simulink model "Final_Model_Project1"  (R2023b)
settings: Solver=ode4  StartTime=0.0  StopTime=2  FixedStep=2e-6  RelTol=1e-3
values from neighbouring files (symbols this model uses):
  C1 = 0.7029    [Fixed_Speed_Wind_Turbine.m]
  C2 = 116.055    [Fixed_Speed_Wind_Turbine.m]
  C3 = 0.4    [Fixed_Speed_Wind_Turbine.m]
  C4 = 0    [Fixed_Speed_Wind_Turbine.m]
  C5 = 8.6614    [Fixed_Speed_Wind_Turbine.m]
  C6 = 21.5    [Fixed_Speed_Wind_Turbine.m]
  C7 = 0.00684    [Fixed_Speed_Wind_Turbine.m]
  Fg = 50    [Fixed_Speed_Wind_Turbine.m]
  Fs = 50    [Fixed_Speed_Wind_Turbine.m]
  J = 1200    [Fixed_Speed_Wind_Turbine.m]
  Llr = 0.06492e-3    (= 6.492e-05)    [Fixed_Speed_Wind_Turbine.m]
  Lls = 0.06492e-3    (= 6.492e-05)    [Fixed_Speed_Wind_Turbine.m]
  optical_tsr_value = (n_mr*(2*pi/60)*r_t)/v_wr    (= 6.49262481742)    [Fixed_Speed_Wind_Turbine.m]
  P = 2    [Fixed_Speed_Wind_Turbine.m]
  p_row = 1.225    [Fixed_Speed_Wind_Turbine.m]
  Ps = (2.3e6)    (= 2300000)    [Fixed_Speed_Wind_Turbine.m]
  r_t = 46.5    [Fixed_Speed_Wind_Turbine.m]
  rgb = 94.5    [Fixed_Speed_Wind_Turbine.m]
  Rr = 1.497e-3    (= 0.001497)    [Fixed_Speed_Wind_Turbine.m]
  Rs = 1.102e-3    (= 0.001102)    [Fixed_Speed_Wind_Turbine.m]
  slip = (nsyn-nmInit)/nsyn    (= 0.0333333333333)    [Fixed_Speed_Wind_Turbine.m]
  SR = 2.59e6    (= 2590000)    [Fixed_Speed_Wind_Turbine.m]
  VgLL = 690    [Fixed_Speed_Wind_Turbine.m]
  VsLL = 690    [Fixed_Speed_Wind_Turbine.m]
libraries: spsAsynchronousMachineSIUnitsLib x1, spsThreePhaseVIMeasurementLib x1, slpidlib x1, spsPower3phInstantaneousLib x1, spsGroundLib x1, spsThreePhaseProgrammableVoltageSourceLib x1, simulink x1, sps_lib x1
settings Model: Creator=priya  LastModifiedBy=priya
settings SolverCC: AutoInsertRateTranBlk=on

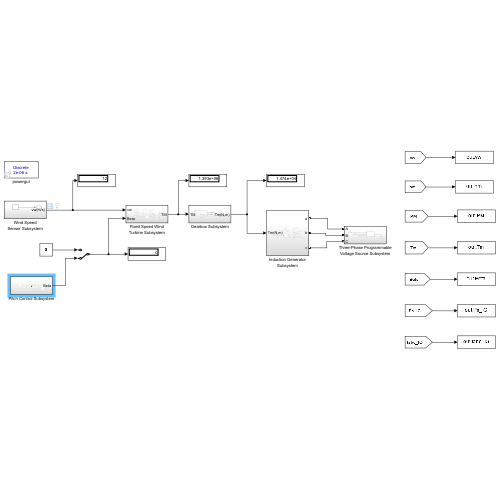
[thumbnail: Simulink's stored preview of the top-level diagram]
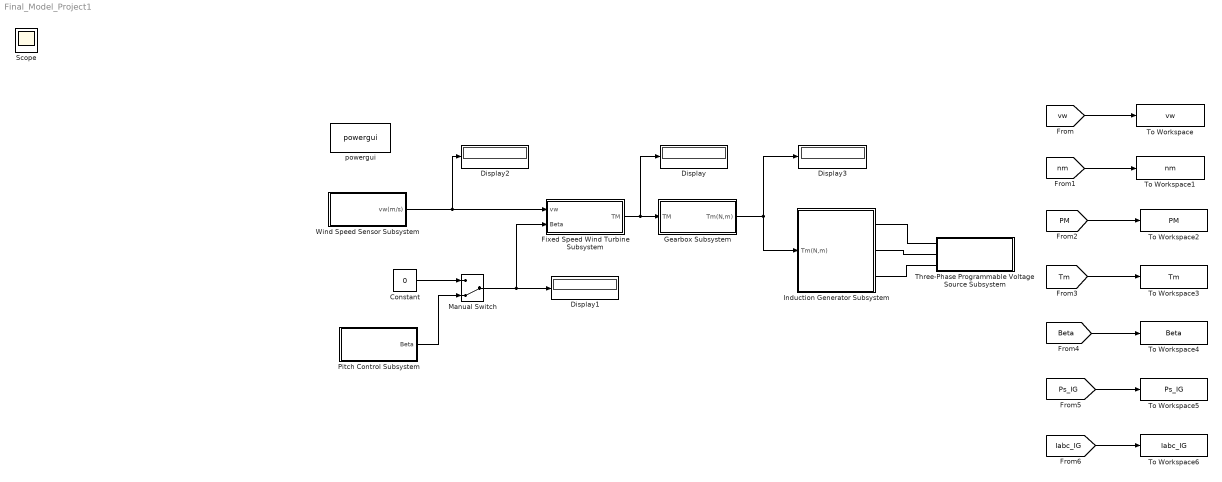
== system Final_Model_Project1 ==
  Constant : Constant  Value=0
  Display{,1..3} (4 alike) : Display
  Fixed Speed Wind Turbine Subsystem : Subsystem
  Gearbox Subsystem : Subsystem
  Induction Generator Subsystem : Subsystem
  Manual Switch : ManualSwitch  CurrentSetting=0
  Pitch Control Subsystem : Subsystem
  Three-Phase Programmable Voltage Source Subsystem : Subsystem
  To Workspace : ToWorkspace  VariableName=vw  SampleTime=-1
  To Workspace1 : ToWorkspace  VariableName=nm  SampleTime=-1
  To Workspace2 : ToWorkspace  VariableName=PM  SampleTime=-1
  To Workspace3 : ToWorkspace  VariableName=Tm  SampleTime=-1
  To Workspace4 : ToWorkspace  VariableName=Beta  SampleTime=-1
  To Workspace5 : ToWorkspace  VariableName=Ps_IG  SampleTime=-1
  To Workspace6 : ToWorkspace  VariableName=Iabc_IG  SampleTime=-1
  Wind Speed Sensor Subsystem : Subsystem
  powergui : sps_lib/powergui  Priority=1  SimulationMode=Discrete  SampleTime=2e-6  frequency=60  Iterations=50  frequencyindice=50  Pbase=100e6  ErrMax=1e-4  UnitsV=kV  UnitsW=MW  buscounter=0  FunctionMessages=off  echomessages=off  EnableUseOfTLC=off  CurrentSourceSwitches=off  DisableSnubberDevices=off  DisableRonSwitches=off  DisableVfSwitches=off  DisplayEquations=off  AutomaticDiscreteSolvers=off  SolverType=Tustin/Backward Euler (TBE)  Interpol=off  ExternalGateDelay=off  methode=off  Ts=100  x0status=blocks  SPID=on  SwTol=0  HookPort=off  NonlinearTolerance=1e-4  nMaxIteration=100  ContinueOnMaxIteration=off  RestoreLinks=warning  ResistiveCurrentMeasurement=off  Frange=[0:2:500]  Ylog=off  Xlog=on  ShowGrid=off  save=off  variable=ZData  structure=0  ZoomFFT=off  StartTime=0.0  cycles=1  DisplayStyle=1  fundamental=60  FreqAxis=off  MaxFrequency=1000  frequencyindicesteady=1  RmsSteady=1  display=off
  Scope : Scope
  wires:
  Gearbox Subsystem/1(Tm(N,m)) -> Display3/1, Induction Generator Subsystem/1(Tm(N,m))
  Pitch Control Subsystem/1(Beta) -> Manual Switch/2
  Fixed Speed Wind Turbine Subsystem/1(TM) -> Display/1, Gearbox Subsystem/1(TM)
  Manual Switch/1 -> Display1/1, Fixed Speed Wind Turbine Subsystem/2(Beta)
  Constant/1 -> Manual Switch/1
  Wind Speed Sensor Subsystem/1(vw(m/s)) -> Display2/1, Fixed Speed Wind Turbine Subsystem/1(vw)
  [vw] -> To Workspace/1
  [nm] -> To Workspace1/1
  [PM] -> To Workspace2/1
  [Tm] -> To Workspace3/1
  [Beta] -> To Workspace4/1
  [Ps_IG] -> To Workspace5/1
  [Iabc_IG] -> To Workspace6/1
  connections:
  Three-Phase Programmable Voltage Source Subsystem/LConn1 -- Induction Generator Subsystem/RConn1
  Three-Phase Programmable Voltage Source Subsystem/LConn2 -- Induction Generator Subsystem/RConn2
  Three-Phase Programmable Voltage Source Subsystem/LConn3 -- Induction Generator Subsystem/RConn3

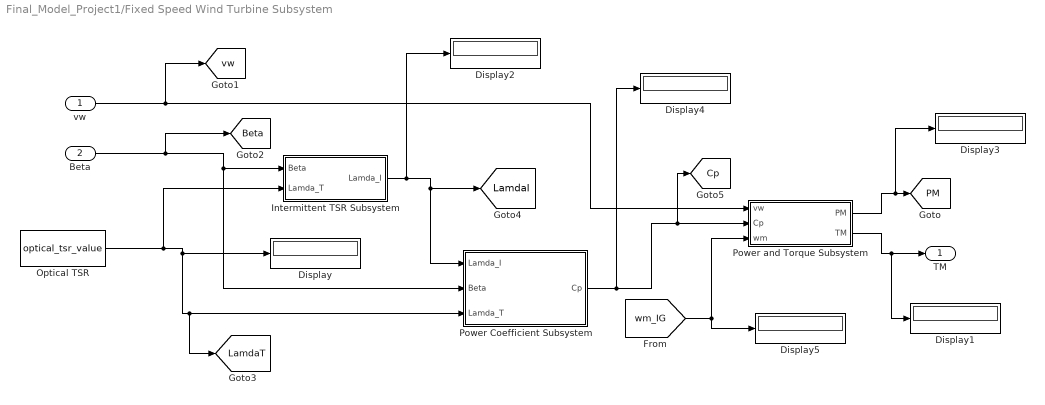
== system Final_Model_Project1/Fixed Speed Wind Turbine Subsystem ==
  vw : Inport
  Beta : Inport  Port=2
  Display{,1..5} (6 alike) : Display
  Intermittent TSR Subsystem : Subsystem
  Optical TSR : Constant  Value=optical_tsr_value
  Power Coefficient Subsystem : Subsystem
  Power and Torque Subsystem : Subsystem
  TM : Outport
  tag scope: Beta=global, Cp=global, LamdaI=global, LamdaT=global, PM=global, vw=global
  wires:
  Power and Torque Subsystem/1(PM) -> Display3/1, [PM]
  Power and Torque Subsystem/2(TM) -> Display1/1, TM/1
  Power Coefficient Subsystem/1(Cp) -> Display4/1, [Cp], Power and Torque Subsystem/2(Cp)
  Optical TSR/1 -> Intermittent TSR Subsystem/2(Lamda_T), [LamdaT], Power Coefficient Subsystem/3(Lamda_T), Display/1
  Beta/1 -> [Beta], Intermittent TSR Subsystem/1(Beta), Power Coefficient Subsystem/2(Beta)
  Intermittent TSR Subsystem/1(Lamda_I) -> Display2/1, Power Coefficient Subsystem/1(Lamda_I), [LamdaI]
  vw/1 -> [vw], Power and Torque Subsystem/1(vw)
  [wm_IG] -> Display5/1, Power and Torque Subsystem/3(wm)

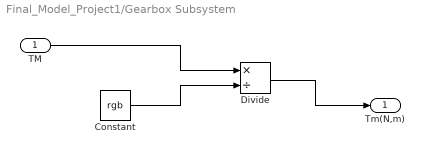
== system Final_Model_Project1/Gearbox Subsystem ==
  TM : Inport
  Constant : Constant  Value=rgb
  Divide : Product  Inputs=*/
  Tm(N,m) : Outport
  wires:
  TM/1 -> Divide/1
  Constant/1 -> Divide/2
  Divide/1 -> Tm(N,m)/1

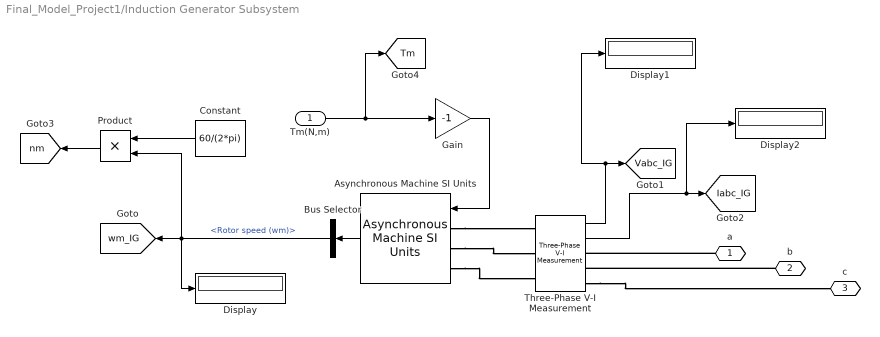
== system Final_Model_Project1/Induction Generator Subsystem ==
  Tm(N,m) : Inport
  Asynchronous Machine SI Units : spsAsynchronousMachineSIUnitsLib/Asynchronous Machine SI Units  RotorType=Squirrel-cage  PresetModel=No  MechanicalLoad=Torque Tm  ShowDetailedParameters=on  ReferenceFrame=Stationary  Units=SI  MeasurementBus=off  NominalParameters="[SR  VsLL Fs]"  VoltageRatio=1  Stator=[Rs Lls]  Rotor=[Rr Llr]  Cage1=[0.4155 0.002066]  Cage2=[0.4168 0.0003495]  Lm=Lm  Mechanical=[J 0 P]  PolePairs=2  InitialConditions=[slip 0 0 0 0 0 0 0]  SimulateSaturation=off  Saturation=[14.03593122, 27.81365428, 53.79336849, 72.68890987, 97.98006896, 148.6815601, 215.7428561, 302.9841135, 428.7778367 ; 230, 322, 414, 460, 506, 552, 598, 644, 690]  LoadFlowParameters=1492000  TsPowergui=0  TsBlock=-1  IterativeModel=Trapezoidal non iterative  IterativeDiscreteModel=Trapezoidal non iterative  Pmec=1.492e+006
  Bus Selector : BusSelector  OutputSignals=Mechanical.Rotor speed (wm)
  Constant : Constant  Value=60/(2*pi)
  Display : Display
  Display1 : Display
  Display2 : Display
  Gain : Gain  Gain=-1
  Product : Product
  Three-Phase V-I Measurement : spsThreePhaseVIMeasurementLib/Three-Phase V-I Measurement  VoltageMeasurement=phase-to-ground  SetLabelV=off  LabelV=Vabc_IG  Vpu=off  VpuLL=off  CurrentMeasurement=yes  SetLabelI=off  LabelI=Iabc_IG  Ipu=off  Pbase=100e6  Vbase=500e3  OutputType=Complex  PhasorSimulation=off  PSBequivalent=0
  a : PMIOPort  Side=Right
  b : PMIOPort  Port=2  Side=Right
  c : PMIOPort  Port=3  Side=Right
  tag scope: Iabc_IG=global, Tm=global, Vabc_IG=global, nm=global, wm_IG=global
  wires:
  Asynchronous Machine SI Units/1 -> Bus Selector/1
  Tm(N,m)/1 -> [Tm], Gain/1
  Gain/1 -> Asynchronous Machine SI Units/1
  Bus Selector/1 -> Product/2, Display/1, [wm_IG]  "<Rotor speed (wm)>"
  Three-Phase V-I Measurement/1 -> Display1/1, [Vabc_IG]
  Three-Phase V-I Measurement/2 -> Display2/1, [Iabc_IG]
  Constant/1 -> Product/1
  Product/1 -> [nm]
  connections:
  Asynchronous Machine SI Units/LConn1 -- Three-Phase V-I Measurement/LConn1
  Asynchronous Machine SI Units/LConn2 -- Three-Phase V-I Measurement/LConn2
  Asynchronous Machine SI Units/LConn3 -- Three-Phase V-I Measurement/LConn3
  Three-Phase V-I Measurement/RConn3 -- c/RConn1
  b/RConn1 -- Three-Phase V-I Measurement/RConn2
  a/RConn1 -- Three-Phase V-I Measurement/RConn1

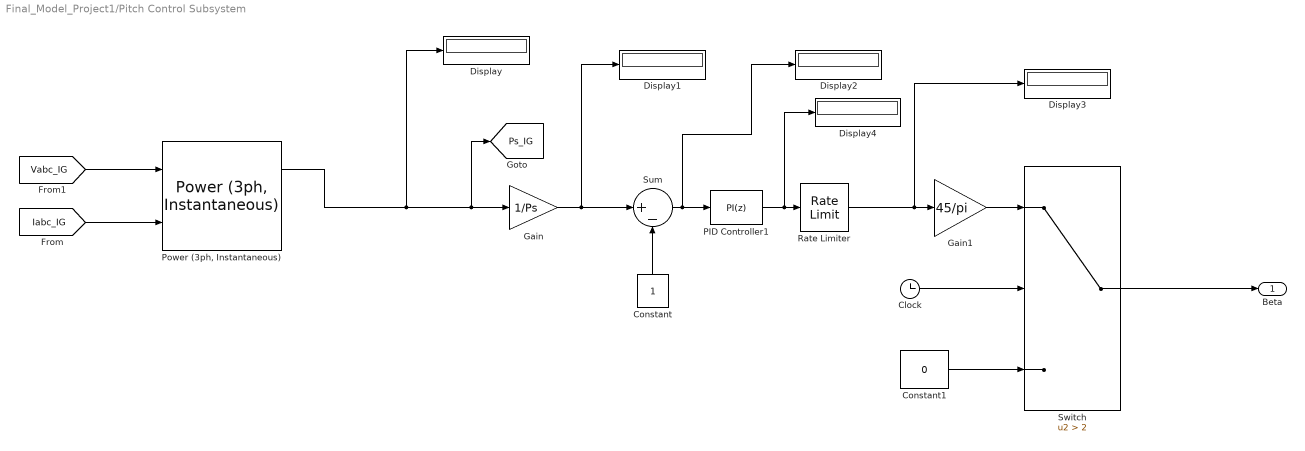
== system Final_Model_Project1/Pitch Control Subsystem ==
  Clock : Clock
  Constant : Constant
  Constant1 : Constant  Value=0
  Display{,1..4} (5 alike) : Display
  Gain : Gain  Gain=1/Ps
  Gain1 : Gain  Gain=45/pi
  PID Controller1 : slpidlib/PID Controller  Controller=PI  Form=Parallel  TimeDomain=Discrete-time  UseExternalTs=off  SampleTime=2e-6  IntegratorMethod=Forward Euler  FilterMethod=Forward Euler  ControllerParametersSource=internal  P=100  I=0.001  UseKiTs=off  D=0  N=100  UseFilter=on  TunerSelectOption=Transfer Function Based (PID Tuner App)  InitialConditionSource=internal  InitialConditionForIntegrator=0  InitialConditionForFilter=0  DifferentiatorICPrevScaledInput=0  ExternalReset=none  TrackingMode=off  Kt=1  LimitOutput=on  SatLimitsSource=internal  UpperSaturationLimit=45  LowerSaturationLimit=0  LinearizeAsGain=on  AntiWindupMode=none  Kb=1  LimitIntegrator=off  UpperIntegratorSaturationLimit=inf  LowerIntegratorSaturationLimit=-inf  POutMin=[]  POutMax=[]  IOutMin=[]  IOutMax=[]  DOutMin=[]  DOutMax=[]  NOutMin=[]  NOutMax=[]  SumOutMin=[]  SumOutMax=[]  SaturationOutMin=[]  SaturationOutMax=[]  PParamMin=[]  PParamMax=[]  IParamMin=[]  IParamMax=[]  DParamMin=[]  DParamMax=[]  NParamMin=[]  NParamMax=[]  KbParamMin=[]  KbParamMax=[]  KtParamMin=[]  KtParamMax=[]  KbOutMin=[]  KbOutMax=[]  KtOutMin=[]  KtOutMax=[]  IntegratorOutMin=[]  IntegratorOutMax=[]  FilterOutMin=[]  FilterOutMax=[]  SumI1OutMin=[]  SumI1OutMax=[]  SumI2OutMin=[]  SumI2OutMax=[]  SumI3OutMin=[]  SumI3OutMax=[]  SumI4OutMin=[]  SumI4OutMax=[]  SumDOutMin=[]  SumDOutMax=[]  DifferentiatorOutMin=[]  DifferentiatorOutMax=[]  FilterDiffOutCoefMin=[]  FilterDiffOutCoefMax=[]  ReciprocalOutMin=[]  ReciprocalOutMax=[]  SumDenOutMin=[]  SumDenOutMax=[]  SumNumOutMin=[]  SumNumOutMax=[]  DivideOutMin=[]  DivideOutMax=[]  UdiffTsProdOutMin=[]  UdiffTsProdOutMax=[]  NTsProdOutMin=[]  NTsProdOutMax=[]  UintegralTsProdOutMin=[]  UintegralTsProdOutMax=[]  UngainTsProdOutMin=[]  UngainTsProdOutMax=[]  ClampingZeroOutDataTypeStr=Inherit: Inherit via back propagation  ClampingZeroOutMin=[]  ClampingZeroOutMax=[]  FilterDenConstantOutDataTypeStr=Inherit: Inherit via back propagation  FilterDenConstantOutMin=[]  FilterDenConstantOutMax=[]  PCopyOutDataTypeStr=Inherit: Inherit via back propagation  PCopyOutMin=[]  PCopyOutMax=[]  NCopyOutDataTypeStr=Inherit: Inherit via back propagation  NCopyOutMin=[]  NCopyOutMax=[]  IntegratorContinuousStateAttributes=''  IntegratorStateMustResolveToSignalObject=off  IntegratorRTWStateStorageClass=Auto  FilterContinuousStateAttributes=''  FilterStateMustResolveToSignalObject=off  FilterRTWStateStorageClass=Auto  ParallelPVariant=InternalParameters  IdealPVariant=Disabled  IVariant=InternalParameters  DVariant=Disabled  IntegratorVariant=Discrete  SatVariant=Enabled  AWVariant=Passthrough  PCopyVariant=Disabled  TRVariant=Disabled  FdbkBlocksVariant=Forward  IdealPFdbkVariant=Disabled  SatFdbkVariant=Disabled  DerivativeFilterVariant=Disabled  NVariant=Disabled  NCopyVariant=Disabled_SignalSpec  FilterICVariant=Disabled  IntegratorICVariant=InternalICs  ExternalResetVariant=Disabled  TRSumVariant=Passthrough  SumFdbkVariant=Disabled  SumVariant=Sum_PI  TsampFilterVariant=InternalTs  TsampNgainVariant=Passthrough  TsampIntegralVariant=Disabled_SignalSpec  ExternalSaturationOutDataTypeStr=Inherit: Same as second input
  "Power (3ph, Instantaneous)" : spsPower3phInstantaneousLib/Power (3ph, Instantaneous)
  Rate Limiter : RateLimiter  RisingSlewLimit=10  FallingSlewLimit=-10  SampleTimeMode=inherited
  Sum : Sum  Inputs=|+-
  Switch : Switch  Criteria=u2 > Threshold  Threshold=2  SaturateOnIntegerOverflow=off  InputSameDT=off
  Beta : Outport
  tag scope: Ps_IG=global
  wires:
  [Vabc_IG] -> "Power (3ph, Instantaneous)"/1
  [Iabc_IG] -> "Power (3ph, Instantaneous)"/2
  "Power (3ph, Instantaneous)"/1 -> Display/1, Gain/1, [Ps_IG]
  Constant/1 -> Sum/2
  Rate Limiter/1 -> Display3/1, Gain1/1
  Gain1/1 -> Switch/1
  Clock/1 -> Switch/2
  Constant1/1 -> Switch/3
  Switch/1 -> Beta/1
  Sum/1 -> PID Controller1/1, Display2/1
  Gain/1 -> Display1/1, Sum/1
  PID Controller1/1 -> Display4/1, Rate Limiter/1

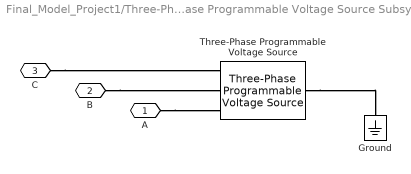
== system Final_Model_Project1/Three-Phase Programmable Voltage Source Subsystem ==
  Ground : spsGroundLib/Ground  LConnTagsString=a
  Three-Phase Programmable Voltage Source : spsThreePhaseProgrammableVoltageSourceLib/Three-Phase Programmable Voltage Source  PositiveSequence=[VgLL 0 Fg]  VariationEntity=None  VariationType=Table of time-amplitude pairs  VariationTypeAlt=Step  VariationStep=0.5  VariationRate=10  VariationMagnitude=0.3  VariationFrequency=2  VariationTiming=[1 2]  VariationPhaseA=off  Amplitudes=[1 0.8 1.2 1.0]  TimeValues=[0 0.1 0.15 0.2]  HarmonicGeneration=off  HarmonicA=[3 0.2 -25 0]  HarmonicB=[2 0.15 35 2]  Timing="[0.05  3]"  BusType=swing  Pref=0  Qref=0  Qmin=-inf  Qmax=inf
  A : PMIOPort  Side=Left
  B : PMIOPort  Port=2  Side=Left
  C : PMIOPort  Port=3  Side=Left
  connections:
  Three-Phase Programmable Voltage Source/LConn1 -- Ground/LConn1
  A/RConn1 -- Three-Phase Programmable Voltage Source/RConn1
  B/RConn1 -- Three-Phase Programmable Voltage Source/RConn2
  C/RConn1 -- Three-Phase Programmable Voltage Source/RConn3

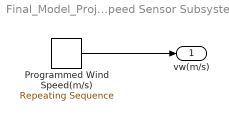
== system Final_Model_Project1/Wind Speed Sensor Subsystem ==
  Programmed Wind Speed(m/s) : simulink/Sources/Repeating Sequence  rep_seq_t=[0 1.2 2.4 2.8 3.2 3.6 5]  rep_seq_y=[0.0001 12 12 15 15 12 12]
  vw(m/s) : Outport
  wires:
  Programmed Wind Speed(m/s)/1 -> vw(m/s)/1

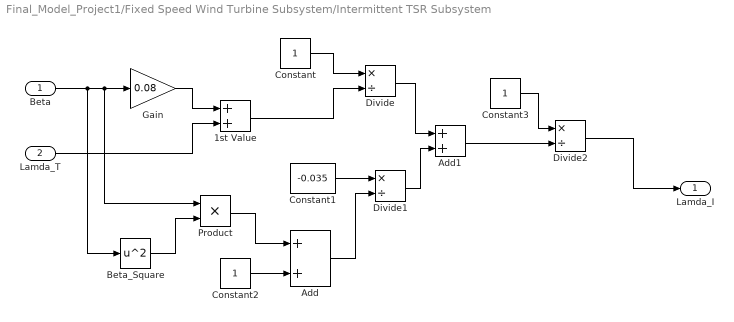
== system Final_Model_Project1/Fixed Speed Wind Turbine Subsystem/Intermittent TSR Subsystem ==
  Beta : Inport
  Lamda_T : Inport  Port=2
  1st Value : Sum
  Add : Sum
  Add1 : Sum
  Beta_Square : Math  Operator=square
  Constant : Constant
  Constant1 : Constant  Value=-0.035
  Constant2 : Constant
  Constant3 : Constant
  Divide : Product  Inputs=*/
  Divide1 : Product  Inputs=*/
  Divide2 : Product  Inputs=*/
  Gain : Gain  Gain=0.08
  Product : Product
  Lamda_I : Outport
  wires:
  Beta/1 -> Product/1, Gain/1, Beta_Square/1
  Gain/1 -> 1st Value/1
  Lamda_T/1 -> 1st Value/2
  Constant/1 -> Divide/1
  1st Value/1 -> Divide/2
  Beta_Square/1 -> Product/2
  Product/1 -> Add/1
  Constant2/1 -> Add/2
  Constant1/1 -> Divide1/1
  Add/1 -> Divide1/2
  Divide/1 -> Add1/1
  Divide1/1 -> Add1/2
  Add1/1 -> Divide2/2
  Constant3/1 -> Divide2/1
  Divide2/1 -> Lamda_I/1

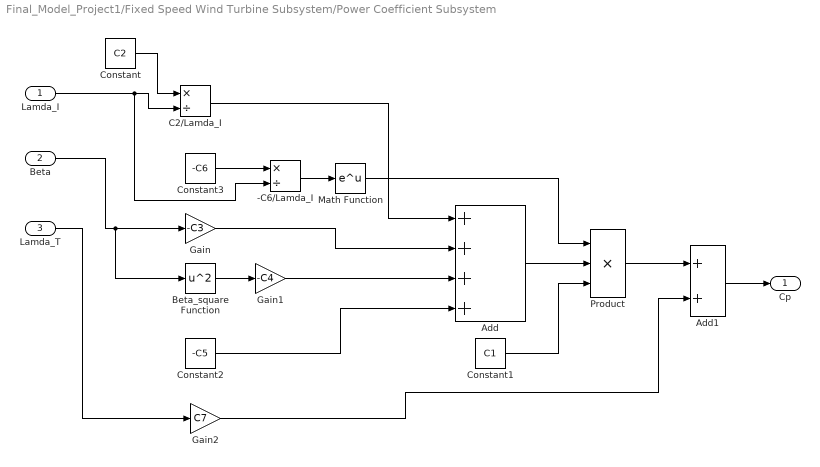
== system Final_Model_Project1/Fixed Speed Wind Turbine Subsystem/Power Coefficient Subsystem ==
  Lamda_I : Inport
  Beta : Inport  Port=2
  Lamda_T : Inport  Port=3
  -C6/Lamda_I : Product  Inputs=*/
  Add : Sum  Inputs=++++
  Add1 : Sum
  Beta_square Function : Math  Operator=square
  C2/Lamda_I : Product  Inputs=*/
  Constant : Constant  Value=C2
  Constant1 : Constant  Value=C1
  Constant2 : Constant  Value=-C5
  Constant3 : Constant  Value=-C6
  Gain : Gain  Gain=-C3
  Gain1 : Gain  Gain=-C4
  Gain2 : Gain  Gain=C7
  Math Function : Math
  Product : Product  Inputs=3
  Cp : Outport
  wires:
  Lamda_I/1 -> -C6/Lamda_I/2, C2/Lamda_I/2
  Constant/1 -> C2/Lamda_I/1
  Beta/1 -> Beta_square Function/1, Gain/1
  Beta_square Function/1 -> Gain1/1
  Lamda_T/1 -> Gain2/1
  Constant3/1 -> -C6/Lamda_I/1
  -C6/Lamda_I/1 -> Math Function/1
  C2/Lamda_I/1 -> Add/1
  Gain/1 -> Add/2
  Gain1/1 -> Add/3
  Constant2/1 -> Add/4
  Add/1 -> Product/2
  Constant1/1 -> Product/3
  Math Function/1 -> Product/1
  Gain2/1 -> Add1/2
  Product/1 -> Add1/1
  Add1/1 -> Cp/1

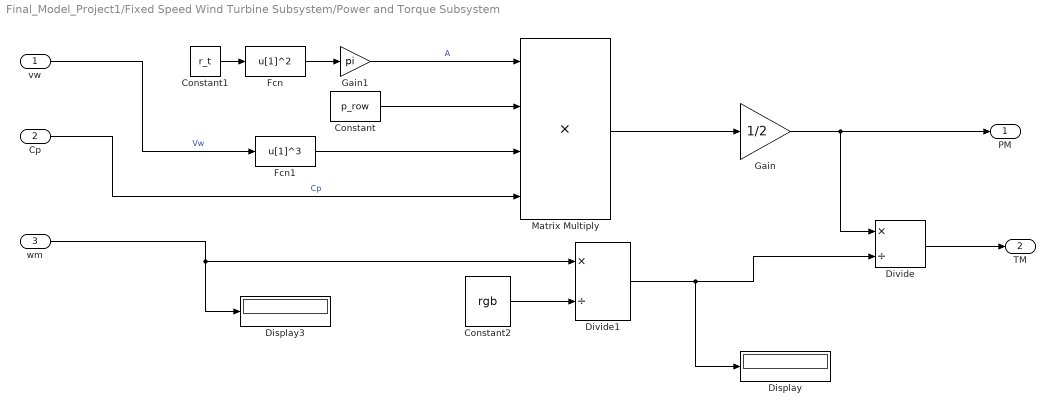
== system Final_Model_Project1/Fixed Speed Wind Turbine Subsystem/Power and Torque Subsystem ==
  vw : Inport
  Cp : Inport  Port=2
  wm : Inport  Port=3
  Constant : Constant  Value=p_row
  Constant1 : Constant  Value=r_t
  Constant2 : Constant  Value=rgb
  Display : Display
  Display3 : Display
  Divide : Product  Inputs=*/
  Divide1 : Product  Inputs=*/
  Fcn : Fcn  Expr=u[1]^2
  Fcn1 : Fcn  Expr=u[1]^3
  Gain : Gain  Gain=1/2
  Gain1 : Gain  Gain=pi
  Matrix Multiply : Product  Inputs=4
  PM : Outport
  TM : Outport  Port=2
  wires:
  Gain1/1 -> Matrix Multiply/1  "A"
  Matrix Multiply/1 -> Gain/1
  Constant/1 -> Matrix Multiply/2
  Cp/1 -> Matrix Multiply/4  "Cp"
  vw/1 -> Fcn1/1  "Vw"
  Fcn/1 -> Gain1/1
  Gain/1 -> Divide/1, PM/1
  Constant1/1 -> Fcn/1
  wm/1 -> Display3/1, Divide1/1
  Divide/1 -> TM/1
  Fcn1/1 -> Matrix Multiply/3
  Constant2/1 -> Divide1/2
  Divide1/1 -> Display/1, Divide/2
